simulink model "test"  (R2016a)
settings: Solver=FixedStepDiscrete  StartTime=0.0  StopTime=10  FixedStep=2.5  RelTol=1e-3
settings Model: Creator=Simon_Zhong  LastModifiedBy=SimonLaplace

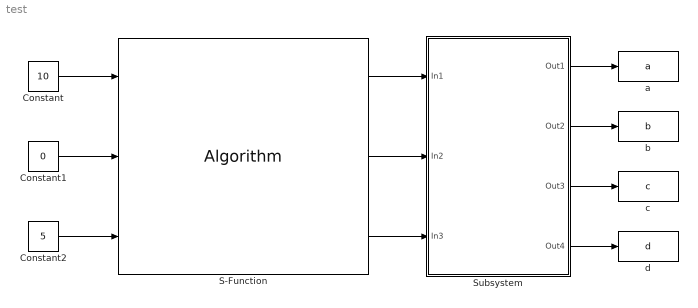
== system test ==
  Constant : Constant  Value=10
  Constant1 : Constant  Value=0
  Constant2 : Constant  Value=5
  S-Function : S-Function  FunctionName=Algorithm  SFunctionDeploymentMode=off  EnableBusSupport=off
  Subsystem : Subsystem
  a : ToWorkspace  VariableName=a  SaveFormat=Timeseries  SampleTime=-1
  b : ToWorkspace  VariableName=b  SaveFormat=Timeseries  SampleTime=-1
  c : ToWorkspace  VariableName=c  SaveFormat=Timeseries  SampleTime=-1
  d : ToWorkspace  VariableName=d  SaveFormat=Timeseries  SampleTime=-1
  wires:
  Constant/1 -> S-Function/1
  Constant2/1 -> S-Function/3
  Constant1/1 -> S-Function/2
  S-Function/1 -> Subsystem/1(In1)
  S-Function/2 -> Subsystem/2(In2)
  S-Function/3 -> Subsystem/3(In3)
  Subsystem/1(Out1) -> a/1
  Subsystem/2(Out2) -> b/1
  Subsystem/3(Out3) -> c/1
  Subsystem/4(Out4) -> d/1

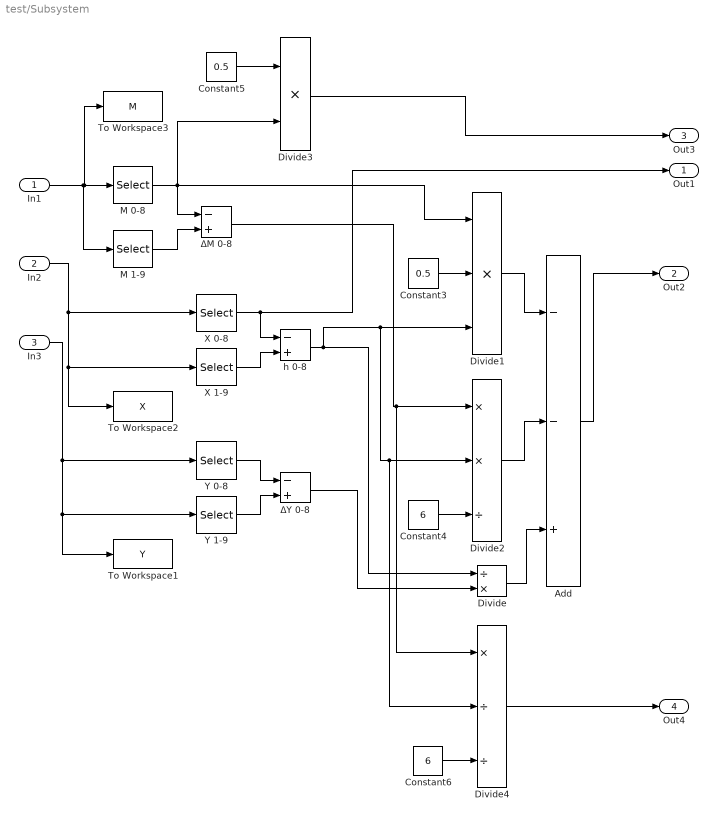
== system test/Subsystem ==
  In1 : Inport
  In2 : Inport  Port=2
  In3 : Inport  Port=3
  Add : Sum  Inputs=--+
  Constant3 : Constant  Value=0.5
  Constant4 : Constant  Value=6
  Constant5 : Constant  Value=0.5
  Constant6 : Constant  Value=6
  Divide : Product  Inputs=/*
  Divide1 : Product  Inputs=***
  Divide2 : Product  Inputs=**/
  Divide3 : Product  Inputs=**
  Divide4 : Product  Inputs=*//
  M 0-8 : Selector  InputPortWidth=10  IndexOptions=Index vector (dialog)  Indices=[1 2 3 4 5 6 7 8 9]  OutputSizes=1
  M 1-9 : Selector  InputPortWidth=10  IndexOptions=Index vector (dialog)  Indices=[2 3 4 5 6 7 8 9 10]  OutputSizes=1
  To Workspace1 : ToWorkspace  VariableName=Y  SaveFormat=Timeseries  SampleTime=-1
  To Workspace2 : ToWorkspace  VariableName=X  SaveFormat=Timeseries  SampleTime=-1
  To Workspace3 : ToWorkspace  VariableName=M  SaveFormat=Timeseries  SampleTime=-1
  X 0-8 : Selector  InputPortWidth=10  IndexOptions=Index vector (dialog)  Indices=[1 2 3 4 5 6 7 8 9]  OutputSizes=1
  X 1-9 : Selector  InputPortWidth=10  IndexOptions=Index vector (dialog)  Indices=[2 3 4 5 6 7 8 9 10]  OutputSizes=1
  Y 0-8 : Selector  InputPortWidth=10  IndexOptions=Index vector (dialog)  Indices=[1 2 3 4 5 6 7 8 9]  OutputSizes=1
  Y 1-9 : Selector  InputPortWidth=10  IndexOptions=Index vector (dialog)  Indices=[2 3 4 5 6 7 8 9 10]  OutputSizes=1
  h 0-8 : Sum  Inputs=-+
  ΔM 0-8 : Sum  Inputs=-+
  ΔY 0-8 : Sum  Inputs=-+
  Out1 : Outport
  Out2 : Outport  Port=2
  Out3 : Outport  Port=3
  Out4 : Outport  Port=4
  wires:
  X 0-8/1 -> Out1/1, h 0-8/1
  X 1-9/1 -> h 0-8/2
  Divide3/1 -> Out3/1
  Y 1-9/1 -> ΔY 0-8/2
  Y 0-8/1 -> ΔY 0-8/1
  ΔY 0-8/1 -> Divide/2
  In3/1 -> Y 0-8/1, Y 1-9/1, To Workspace1/1
  Constant5/1 -> Divide3/1
  M 1-9/1 -> ΔM 0-8/2
  In2/1 -> X 0-8/1, To Workspace2/1, X 1-9/1
  In1/1 -> M 1-9/1, To Workspace3/1, M 0-8/1
  ΔM 0-8/1 -> Divide4/1, Divide2/1
  Divide/1 -> Add/3
  Constant3/1 -> Divide1/2
  Constant4/1 -> Divide2/3
  Divide1/1 -> Add/1
  Add/1 -> Out2/1
  Constant6/1 -> Divide4/3
  Divide4/1 -> Out4/1
  h 0-8/1 -> Divide/1, Divide4/2, Divide2/2, Divide1/3
  M 0-8/1 -> Divide3/2, Divide1/1, ΔM 0-8/1
  Divide2/1 -> Add/2
